simulink model "radar_final_cs_old"  (R2019a)
settings: Solver=ode5  StartTime=0.0  StopTime=2  FixedStep=1/20  RelTol=1e-3
PreLoadFcn:
  | mbxruntime.callbacks.PreLoadFcn(bdroot);
PostLoadFcn:
  | mbxruntime.callbacks.PostLoadFcn(bdroot);
InitFcn:
  | mbxruntime.callbacks.InitFcn(bdroot);
StartFcn:
  | mbxruntime.callbacks.StartFcn(bdroot);
StopFcn:
  | mbxruntime.callbacks.StopFcn(bdroot);
model workspace: external: MAT-File .\radar_final_cs_hws.mat (data not in the file)
undefined symbols (not defined in the file or in its folder): Data, Data_SL_Info, DiscIntNeverNeededParam, mbxruntime, radar_final_cs_06f3e03c41833990, radar_final_cs_0ae852e737f0605d, radar_final_cs_2161ee680ff58ba6, radar_final_cs_2267e09559a0c517, radar_final_cs_25fb437f13dc4ac4, radar_final_cs_2a9ff95eb5b29c63, radar_final_cs_2b3b1caad78d25a0, radar_final_cs_36e6d5e535f2778e, radar_final_cs_3f094c3a86d4ef6f, radar_final_cs_414d34a7c1c059ce, radar_final_cs_42788e9f25b76679, radar_final_cs_4442007d7943b1b9, radar_final_cs_57cb0909d4e1963a, radar_final_cs_647e288b34857263, radar_final_cs_7d2d9604fce16766, radar_final_cs_898d5fa4c0c4dce2, radar_final_cs_a56cd948251ec351, radar_final_cs_Audi_A3_2_Path_pathUniqueID, radar_final_cs_Audi_A3_2_SpeedProfile_speedProfileUniqueID, radar_final_cs_bc1d53445e794831, radar_final_cs_bc84f0b4aab11bdd, radar_final_cs_bd2c14ed7a8a21e4, radar_final_cs_bdb595cdc91a90da, radar_final_cs_Boy_150_1_Dynamics_Empty_STATE_Boy_150_1_Pitch0, radar_final_cs_Boy_150_1_Dynamics_Empty_STATE_Boy_150_1_Roll0, radar_final_cs_Boy_150_1_Dynamics_Empty_STATE_Boy_150_1_x0, radar_final_cs_Boy_150_1_Dynamics_Empty_STATE_Boy_150_1_y0, radar_final_cs_Boy_150_1_Dynamics_Empty_STATE_Boy_150_1_Yaw0, radar_final_cs_Boy_150_1_Dynamics_Empty_STATE_Boy_150_1_z0, radar_final_cs_c30ea0c83d921ad6, radar_final_cs_c7f661c76d99b58c, radar_final_cs_ce7e016dbedf2c74, radar_final_cs_cf2ef22c3980d47c, radar_final_cs_d0ac9bfbee56c7a8, radar_final_cs_d13fb20b651cdee7, radar_final_cs_da52fa0c45f9873a, radar_final_cs_f7605f9552b276d3, radar_final_cs_ff9f13297006dd64, radar_final_cs_Skywell_1_Path_pathUniqueID, radar_final_cs_Skywell_1_SpeedProfile_speedProfileUniqueID, tabledata, X, Y
libraries: PreScanSimulinkLibrary x12, simulink x7, robotlib x5, PreScanUsefulBlocks x1
(part 3 of 5)

== system radar_final_cs_old/STATE_Male_Female_HandInHand_1_bus ==
  STATE_Male_Female_HandInHand_1_bus : Inport  Tag=inport/StatePort  OutDataTypeStr=Bus: PRESCAN_STATEACTUATORDATA  PortDimensions=1  SampleTime=1/20  BusOutputAsStruct=on
  Actuator : S-Function  FunctionName=sfun_StateActuator  Parameters=mbxruntime.parameters.convert(UniqueID), mbxruntime.parameters.convert(TimeStep)  SFunctionDeploymentMode=off  EnableBusSupport=off  mask(PreScan Sink Block: State){UniqueID=523, TimeStep=1/20}
      mask prompts: UniqueID "Auto-Assigned: Unique ID"; TimeStep "Auto-Assigned: Upload Period [s]"
      mask help:
      | The Actor State contains a vector signal of size (9x1), containing the following signals:
      |
      | -  Position    	(x,y,z)             	[m]
      | -  Velocity    	(vx,vy,vz)         	[m/s]
      | -  Angles       	(Roll, Pitch, Yaw)	[rad]
      |
      | The Actor state is defined in the global axis system.
      | The state is superponed on the Initial position defined in the GUI.
      |
      | For more information, please click Help.
      mask Help: eval('openHelp(222)')
      mask Display: image(imread('State.png'))
  wires:
  STATE_Male_Female_HandInHand_1_bus/1 -> Actuator/1

== system radar_final_cs_old/STATE_Skywell_1_bus ==
  STATE_Skywell_1_bus : Inport  Tag=inport/StatePort  OutDataTypeStr=Bus: PRESCAN_STATEACTUATORDATA  PortDimensions=1  SampleTime=1/20  BusOutputAsStruct=on
  Actuator : S-Function  FunctionName=sfun_StateActuator  Parameters=mbxruntime.parameters.convert(UniqueID), mbxruntime.parameters.convert(TimeStep)  SFunctionDeploymentMode=off  EnableBusSupport=off  mask(PreScan Sink Block: State){UniqueID=169, TimeStep=1/20}
      mask prompts: UniqueID "Auto-Assigned: Unique ID"; TimeStep "Auto-Assigned: Upload Period [s]"
      mask help:
      | The Actor State contains a vector signal of size (9x1), containing the following signals:
      |
      | -  Position    	(x,y,z)             	[m]
      | -  Velocity    	(vx,vy,vz)         	[m/s]
      | -  Angles       	(Roll, Pitch, Yaw)	[rad]
      |
      | The Actor state is defined in the global axis system.
      | The state is superponed on the Initial position defined in the GUI.
      |
      | For more information, please click Help.
      mask Help: eval('openHelp(222)')
      mask Display: image(imread('State.png'))
  wires:
  STATE_Skywell_1_bus/1 -> Actuator/1

== system radar_final_cs_old/ScenarioEngine ==
  Clock1 : Clock
  Stop Simulation : Stop
  sfun_ScenarioEngine1 : S-Function  FunctionName=sfun_ScenarioEngine  Parameters=TimeStep  SFunctionDeploymentMode=off  EnableBusSupport=off
  wires:
  sfun_ScenarioEngine1/1 -> Stop Simulation/1
  Clock1/1 -> sfun_ScenarioEngine1/1

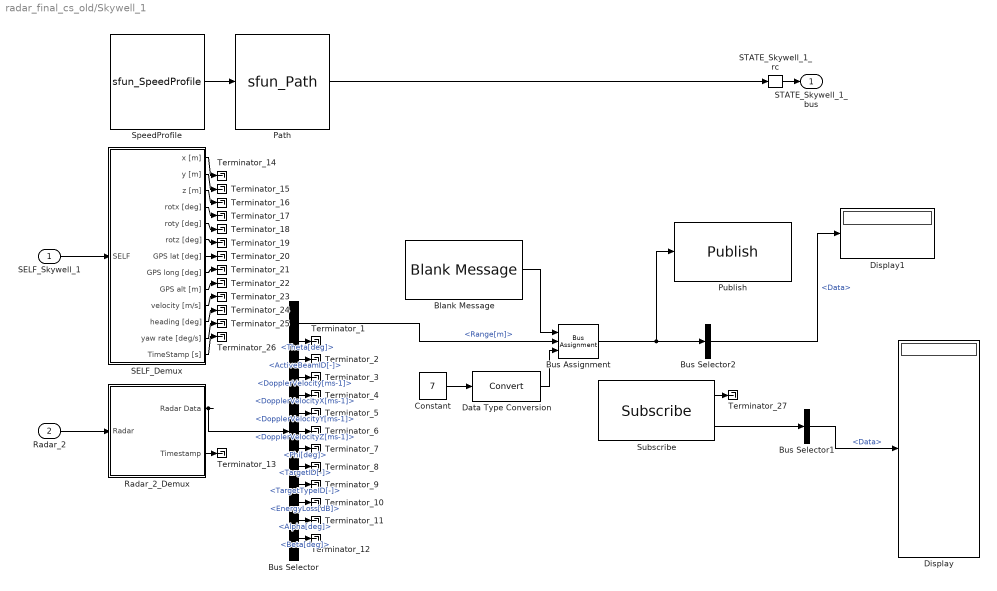
== system radar_final_cs_old/Skywell_1 ==
  SELF_Skywell_1 : Inport  Tag=inport/SelfPort  OutDataTypeStr=Bus: PRESCAN_SELFSENSORDATA  PortDimensions=1  SampleTime=1/20  BusOutputAsStruct=on
  Radar_2 : Inport  Tag=inport/Radar  Port=2  OutDataTypeStr=Bus: PRESCAN_SCANNERSENSOR_MESSAGE  PortDimensions=7  SampleTime=1/4  BusOutputAsStruct=on
  Blank Message : robotlib/Blank Message  messageClass=Message  entityType=std_msgs/Float64MultiArray  messageType=std_msgs/Float64MultiArray  SampleTime=inf
      settings: SourceProductBaseCode=RO
  Bus Assignment : BusAssignment  AssignedSignals=Data,Data_SL_Info.CurrentLength
  Bus Selector : BusSelector  OutputSignals=Range[m],Theta[deg],ActiveBeamID[-],DopplerVelocity[ms-1],DopplerVelocityX[ms-1],DopplerVelocityY[ms-1],DopplerVelocityZ[ms-1],Phi[deg],TargetID[-],TargetTypeID[-],EnergyLoss[dB],Alpha[deg],Beta[deg]
  Bus Selector1 : BusSelector  OutputSignals=Data
  Bus Selector2 : BusSelector  OutputSignals=Data
  Constant : Constant  Value=7
  Data Type Conversion : DataTypeConversion
  Display : Display
  Display1 : Display
  Path : S-Function  LoadFcn=load('PrescanMotionData.mat')  FunctionName=sfun_Path  Parameters=mbxruntime.parameters.convert(uniqueID), pathUniqueID, mbxruntime.parameters.convert(timestep)  SFunctionDeploymentMode=off  EnableBusSupport=off  mask(Path){uniqueID=169, pathUniqueID=radar_final_cs_Skywell_1_Path_pathUniqueID, timestep=1/20}
      mask prompts: uniqueID "Object Unique ID"; pathUniqueID "Path Unique ID"; timestep "MATLAB timestep:"
      mask help:
      | The path block outputs the position along a given trajectory.
      |
      | For more information, please click Help.
      mask Help: eval('openHelp(312)')
      mask Display: image(imread('Path.png'))
  Publish : robotlib/Publish  topicSource=Specify your own  topic=/topic  messageType=std_msgs/Float64MultiArray  messageQueueLength=1
      settings: SourceProductBaseCode=RO
  Radar_2_Demux : Subsystem  Tag=demux/Radar  TreatAsAtomicUnit=on  mask(PreScan Demux Block: Radar){MAXMESSAGES=7}
      mask prompts: MAXMESSAGES "Number of Objects"
      mask help:
      | The Radar Sensor is a detailed sensor based on a physical radar
      | model that includes Antenna GAIN Maps (AGM) and atmospheric
      | attenuation.
      |
      | For more information, please click Help.
      mask Help: eval('openHelp(1464)')
      mask Display:
      | port_label('input',1,'Radar')
      | port_label('output',1,'Radar Data')
      | port_label('output',2,'Timestamp [s]')
  SELF_Demux : Subsystem  Tag=demux/SelfPort  mask(PreScan Demux Block:){}
      mask help:
      | The SELF port shows (state) information of the actor itself. The outputs are position in the experiment's axis system and the GPS coordinates, and the object's absolute velocity and compass heading.
      |
      | For more information, please click Help.
      settings: DeleteFcn=PreScanBlockDeleteFcn;
      mask Help: eval('openHelp(462)')
      mask Display:
      | port_label('output',1,'x [m]')
      | port_label('output',2,'y [m]')
      | port_label('output',3,'z [m]','texmode','on')
      | port_label('output',4,'Rotx [deg]','texmode','on')
      | port_label('output',5,'Roty [deg]','texmode','on')
      | port_label('output',6,'Rotz [deg]','texmode','on')
      | port_label('output',7,'GPS lat [deg]','texmode','on')
      | port_label('output',8,'GPS long [deg]','texmode','on')
      | port_label('output',9,'GPS alt [m]','texmode','on')
      | port_label('output',10,'Velocity [m/s]')
      | port_label('output',11,'Heading [deg]')
      | port_label('output',12,'Yaw rate [deg/s]')
      | port_label('output',13,'Timestamp [s]')
  STATE_Skywell_1_rc : RateTransition  Tag=mux_rc/StatePort  OutPortSampleTimeOpt=Inherit
  SpeedProfile : S-Function  LoadFcn=load('PrescanMotionData.mat')  FunctionName=sfun_SpeedProfile  Parameters=speedProfileUniqueID, mbxruntime.parameters.convert(timestep)  SFunctionDeploymentMode=off  EnableBusSupport=off  mask(SpeedProfile){speedProfileUniqueID=radar_final_cs_Skywell_1_SpeedProfile_speedProfileUniqueID, timestep=1/20}
      mask prompts: speedProfileUniqueID "Speed Profile Unique ID"; timestep "MATLAB timestep:"
      mask help:
      | The speed profile block outputs the travelled distance, velocities and acceleration along a given path.
      |
      | For more information, please click Help.
      mask Help: eval('openHelp(312)')
      mask Display: image(imread('SpeedProfile.png'))
  Subscribe : robotlib/Subscribe  topicSource=Specify your own  topic=/topic  messageType=std_msgs/Float64MultiArray  sampleTime=-1  messageQueueLength=1
      settings: SourceProductBaseCode=RO
  Terminator_{1..27} (27 alike) : Terminator
  STATE_Skywell_1_bus : Outport  Tag=outport/StatePort  OutDataTypeStr=Bus: PRESCAN_STATEACTUATORDATA  PortDimensions=1  SampleTime=1/20
  wires:
  Radar_2_Demux/1(Radar Data) -> Bus Selector/1
  Blank Message/1 -> Bus Assignment/1
  Bus Selector/1 -> Bus Assignment/2  "<Range[m]>"
  Bus Assignment/1 -> Publish/1, Bus Selector2/1
  Subscribe/2 -> Bus Selector1/1
  Bus Selector1/1 -> Display/1  "<Data>"
  Bus Selector2/1 -> Display1/1  "<Data>"
  Data Type Conversion/1 -> Bus Assignment/3
  Constant/1 -> Data Type Conversion/1
  STATE_Skywell_1_rc/1 -> STATE_Skywell_1_bus/1
  SpeedProfile/1 -> Path/1
  Path/1 -> STATE_Skywell_1_rc/1
  SELF_Skywell_1/1 -> SELF_Demux/1(SELF)
  Radar_2/1 -> Radar_2_Demux/1(Radar)
  Bus Selector/2 -> Terminator_1/1  "<Theta[deg]>"
  Bus Selector/3 -> Terminator_2/1  "<ActiveBeamID[-]>"
  Bus Selector/4 -> Terminator_3/1  "<DopplerVelocity[ms-1]>"
  Bus Selector/5 -> Terminator_4/1  "<DopplerVelocityX[ms-1]>"
  Bus Selector/6 -> Terminator_5/1  "<DopplerVelocityY[ms-1]>"
  Bus Selector/7 -> Terminator_6/1  "<DopplerVelocityZ[ms-1]>"
  Bus Selector/8 -> Terminator_7/1  "<Phi[deg]>"
  Bus Selector/9 -> Terminator_8/1  "<TargetID[-]>"
  Bus Selector/10 -> Terminator_9/1  "<TargetTypeID[-]>"
  Bus Selector/11 -> Terminator_10/1  "<EnergyLoss[dB]>"
  Bus Selector/12 -> Terminator_11/1  "<Alpha[deg]>"
  Bus Selector/13 -> Terminator_12/1  "<Beta[deg]>"
  Radar_2_Demux/2(Timestamp) -> Terminator_13/1
  SELF_Demux/1(x [m]) -> Terminator_14/1
  SELF_Demux/2(y [m]) -> Terminator_15/1
  SELF_Demux/3(z [m]) -> Terminator_16/1
  SELF_Demux/4(rotx [deg]) -> Terminator_17/1
  SELF_Demux/5(roty [deg]) -> Terminator_18/1
  SELF_Demux/6(rotz [deg]) -> Terminator_19/1
  SELF_Demux/7(GPS lat [deg]) -> Terminator_20/1
  SELF_Demux/8(GPS long [deg]) -> Terminator_21/1
  SELF_Demux/9(GPS alt [m]) -> Terminator_22/1
  SELF_Demux/10(velocity [m/s]) -> Terminator_23/1
  SELF_Demux/11(heading [deg]) -> Terminator_24/1
  SELF_Demux/12(yaw rate [deg/s]) -> Terminator_25/1
  SELF_Demux/13(TimeStamp [s]) -> Terminator_26/1
  Subscribe/1 -> Terminator_27/1

== system radar_final_cs_old/Synchronizer ==
  Bus Selector1 : BusSelector  OutputSignals=FederateStopped
  Stop Simulation : Stop
  sfun_Synchronizer : S-Function  FunctionName=sfun_Synchronizer  Parameters=SampleTime  SFunctionDeploymentMode=off  EnableBusSupport=off  mask(Legacy Function){SFunctionSpec=void prescan_synchronizer_outputFcn(void ** work1, PRESCAN_SYNCHRONIZEDATA y1[1]), SampleTime=TimeStep, ShowSpec=on}
      mask prompts: SampleTime "Sample time (-1 for inherited):"; ShowSpec "Display function specification"
      mask help:
      | This block allows you to call the legacy functions specified by the following Legacy Code Tool definition:
      | def.SFunctionName = 'sfun_Synchronizer';
      | def.OutputFcnSpec = 'void prescan_synchronizer_outputFcn(void ** work1, PRESCAN_TIMESTAMPDATA u1[1], PRESCAN_SYNCHRONIZEDATA y1[1])';
      | def.StartFcnSpec = 'void prescan_synchronizer_startFcn(void ** work1)';
      | def.TerminateFcnSpec = 'void prescan_synchronizer_terminateFcn(void ** work1)';
      | def.HeaderFiles = {'prescan_synchronizer_data.h'};
      | def.HostLibFiles = {'sensorinterfaced.lib'};
      | def.IncPaths = {'src', 'C:\prescandev\vislibrary\vis\..\pimp\include\sensors\InterfaceRTW'};
      | def.SrcPaths = {'src'};
      | def.LibPaths = {'C:\\prescandev\\vislibrary_build\lib'};
      | def.SampleTime = 'parameterized';
      | def.Options.language = 'C';
      mask Help: <p>This block was generated automatically by the Legacy Code Tool. For detailed help on this tool, call<a href="matlab:legacy_code('help')"> legacy_code('help')</a>.</p>
      mask Callback ShowSpec:
      | if strcmp(get_param(gcbh, 'ShowSpec'), 'on')
      |   set_param(gcbh, 'MaskDisplay', sprintf('fprintf(''%s'');', get_param(gcbh, 'SFunctionSpec')));
      | else
      |   set_param(gcbh, 'MaskDisplay', sprintf('fprintf(''%s'');', get_param(gcbh, 'FunctionName')));
      | end
      mask Display: fprintf('void prescan_synchronizer_outputFcn(void ** work1, PRESCAN_SYNCHRONIZEDATA y1[1])');
  wires:
  sfun_Synchronizer/1 -> Bus Selector1/1
  Bus Selector1/1 -> Stop Simulation/1  "<FederateStopped>"

== system radar_final_cs_old/VISUColorRegion_Lower_Body_Boy_150_1 ==
  VISUColorRegion_Lower_Body_Boy_150_1 : Inport  Tag=inport/ColorRegion  OutDataTypeStr=Bus: PRESCAN_COLOR_DATA  PortDimensions=1  SampleTime=1/20  BusOutputAsStruct=on
  Actuator : S-Function  FunctionName=sfun_ColorActuator  Parameters=mbxruntime.parameters.convert(UniqueID), mbxruntime.parameters.convert(WorldModelSubPath), tabledata, TimeStep  SFunctionDeploymentMode=off  EnableBusSupport=off  mask(PreScan Sink Block: VisuTextureColor){UniqueID=197, WorldModelSubPath=/recolorRegion:name=Lower Body/targetColor, TimeStep=1/20}
      mask prompts: UniqueID "Parent Unique Identifier (auto-generated)"; WorldModelSubPath "WM SubPath(auto-generated)"; TimeStep "Simulink time step"
      mask help:
      | The VisuTextureColor block provides a way to adapt the color of a vehicle.
      |
      | For more information, please click Help.
      mask init:
      | [tabledata] = mbxruntime.parameters.table(UniqueID,WorldModelSubPath);
      mask Help: eval('openHelp(230)')
      mask Display: image(imread('TextureColor.png'))
  wires:
  VISUColorRegion_Lower_Body_Boy_150_1/1 -> Actuator/1

== system radar_final_cs_old/VISUColorRegion_Lower_Body_Child_Leaning_1 ==
  VISUColorRegion_Lower_Body_Child_Leaning_1 : Inport  Tag=inport/ColorRegion  OutDataTypeStr=Bus: PRESCAN_COLOR_DATA  PortDimensions=1  SampleTime=1/20  BusOutputAsStruct=on
  Actuator : S-Function  FunctionName=sfun_ColorActuator  Parameters=mbxruntime.parameters.convert(UniqueID), mbxruntime.parameters.convert(WorldModelSubPath), tabledata, TimeStep  SFunctionDeploymentMode=off  EnableBusSupport=off  mask(PreScan Sink Block: VisuTextureColor){UniqueID=387, WorldModelSubPath=/recolorRegion:name=Lower Body/targetColor, TimeStep=1/20}
      mask prompts: UniqueID "Parent Unique Identifier (auto-generated)"; WorldModelSubPath "WM SubPath(auto-generated)"; TimeStep "Simulink time step"
      mask help:
      | The VisuTextureColor block provides a way to adapt the color of a vehicle.
      |
      | For more information, please click Help.
      mask init:
      | [tabledata] = mbxruntime.parameters.table(UniqueID,WorldModelSubPath);
      mask Help: eval('openHelp(230)')
      mask Display: image(imread('TextureColor.png'))
  wires:
  VISUColorRegion_Lower_Body_Child_Leaning_1/1 -> Actuator/1

== system radar_final_cs_old/VISUColorRegion_Lower_Body_Child_Overweight_1 ==
  VISUColorRegion_Lower_Body_Child_Overweight_1 : Inport  Tag=inport/ColorRegion  OutDataTypeStr=Bus: PRESCAN_COLOR_DATA  PortDimensions=1  SampleTime=1/20  BusOutputAsStruct=on
  Actuator : S-Function  FunctionName=sfun_ColorActuator  Parameters=mbxruntime.parameters.convert(UniqueID), mbxruntime.parameters.convert(WorldModelSubPath), tabledata, TimeStep  SFunctionDeploymentMode=off  EnableBusSupport=off  mask(PreScan Sink Block: VisuTextureColor){UniqueID=388, WorldModelSubPath=/recolorRegion:name=Lower Body/targetColor, TimeStep=1/20}
      mask prompts: UniqueID "Parent Unique Identifier (auto-generated)"; WorldModelSubPath "WM SubPath(auto-generated)"; TimeStep "Simulink time step"
      mask help:
      | The VisuTextureColor block provides a way to adapt the color of a vehicle.
      |
      | For more information, please click Help.
      mask init:
      | [tabledata] = mbxruntime.parameters.table(UniqueID,WorldModelSubPath);
      mask Help: eval('openHelp(230)')
      mask Display: image(imread('TextureColor.png'))
  wires:
  VISUColorRegion_Lower_Body_Child_Overweight_1/1 -> Actuator/1

== system radar_final_cs_old/VISUColorRegion_Lower_Body_Child_Regular_1 ==
  VISUColorRegion_Lower_Body_Child_Regular_1 : Inport  Tag=inport/ColorRegion  OutDataTypeStr=Bus: PRESCAN_COLOR_DATA  PortDimensions=1  SampleTime=1/20  BusOutputAsStruct=on
  Actuator : S-Function  FunctionName=sfun_ColorActuator  Parameters=mbxruntime.parameters.convert(UniqueID), mbxruntime.parameters.convert(WorldModelSubPath), tabledata, TimeStep  SFunctionDeploymentMode=off  EnableBusSupport=off  mask(PreScan Sink Block: VisuTextureColor){UniqueID=389, WorldModelSubPath=/recolorRegion:name=Lower Body/targetColor, TimeStep=1/20}
      mask prompts: UniqueID "Parent Unique Identifier (auto-generated)"; WorldModelSubPath "WM SubPath(auto-generated)"; TimeStep "Simulink time step"
      mask help:
      | The VisuTextureColor block provides a way to adapt the color of a vehicle.
      |
      | For more information, please click Help.
      mask init:
      | [tabledata] = mbxruntime.parameters.table(UniqueID,WorldModelSubPath);
      mask Help: eval('openHelp(230)')
      mask Display: image(imread('TextureColor.png'))
  wires:
  VISUColorRegion_Lower_Body_Child_Regular_1/1 -> Actuator/1

== system radar_final_cs_old/VISUColorRegion_Lower_Body_Child_Regular_2 ==
  VISUColorRegion_Lower_Body_Child_Regular_2 : Inport  Tag=inport/ColorRegion  OutDataTypeStr=Bus: PRESCAN_COLOR_DATA  PortDimensions=1  SampleTime=1/20  BusOutputAsStruct=on
  Actuator : S-Function  FunctionName=sfun_ColorActuator  Parameters=mbxruntime.parameters.convert(UniqueID), mbxruntime.parameters.convert(WorldModelSubPath), tabledata, TimeStep  SFunctionDeploymentMode=off  EnableBusSupport=off  mask(PreScan Sink Block: VisuTextureColor){UniqueID=390, WorldModelSubPath=/recolorRegion:name=Lower Body/targetColor, TimeStep=1/20}
      mask prompts: UniqueID "Parent Unique Identifier (auto-generated)"; WorldModelSubPath "WM SubPath(auto-generated)"; TimeStep "Simulink time step"
      mask help:
      | The VisuTextureColor block provides a way to adapt the color of a vehicle.
      |
      | For more information, please click Help.
      mask init:
      | [tabledata] = mbxruntime.parameters.table(UniqueID,WorldModelSubPath);
      mask Help: eval('openHelp(230)')
      mask Display: image(imread('TextureColor.png'))
  wires:
  VISUColorRegion_Lower_Body_Child_Regular_2/1 -> Actuator/1

== system radar_final_cs_old/VISUColorRegion_Lower_Body_Male_Female_HandInHand_1 ==
  VISUColorRegion_Lower_Body_Male_Female_HandInHand_1 : Inport  Tag=inport/ColorRegion  OutDataTypeStr=Bus: PRESCAN_COLOR_DATA  PortDimensions=1  SampleTime=1/20  BusOutputAsStruct=on
  Actuator : S-Function  FunctionName=sfun_ColorActuator  Parameters=mbxruntime.parameters.convert(UniqueID), mbxruntime.parameters.convert(WorldModelSubPath), tabledata, TimeStep  SFunctionDeploymentMode=off  EnableBusSupport=off  mask(PreScan Sink Block: VisuTextureColor){UniqueID=523, WorldModelSubPath=/recolorRegion:name=Lower Body/targetColor, TimeStep=1/20}
      mask prompts: UniqueID "Parent Unique Identifier (auto-generated)"; WorldModelSubPath "WM SubPath(auto-generated)"; TimeStep "Simulink time step"
      mask help:
      | The VisuTextureColor block provides a way to adapt the color of a vehicle.
      |
      | For more information, please click Help.
      mask init:
      | [tabledata] = mbxruntime.parameters.table(UniqueID,WorldModelSubPath);
      mask Help: eval('openHelp(230)')
      mask Display: image(imread('TextureColor.png'))
  wires:
  VISUColorRegion_Lower_Body_Male_Female_HandInHand_1/1 -> Actuator/1

== system radar_final_cs_old/VISUColorRegion_Shoes_Boy_150_1 ==
  VISUColorRegion_Shoes_Boy_150_1 : Inport  Tag=inport/ColorRegion  OutDataTypeStr=Bus: PRESCAN_COLOR_DATA  PortDimensions=1  SampleTime=1/20  BusOutputAsStruct=on
  Actuator : S-Function  FunctionName=sfun_ColorActuator  Parameters=mbxruntime.parameters.convert(UniqueID), mbxruntime.parameters.convert(WorldModelSubPath), tabledata, TimeStep  SFunctionDeploymentMode=off  EnableBusSupport=off  mask(PreScan Sink Block: VisuTextureColor){UniqueID=197, WorldModelSubPath=/recolorRegion:name=Shoes/targetColor, TimeStep=1/20}
      mask prompts: UniqueID "Parent Unique Identifier (auto-generated)"; WorldModelSubPath "WM SubPath(auto-generated)"; TimeStep "Simulink time step"
      mask help:
      | The VisuTextureColor block provides a way to adapt the color of a vehicle.
      |
      | For more information, please click Help.
      mask init:
      | [tabledata] = mbxruntime.parameters.table(UniqueID,WorldModelSubPath);
      mask Help: eval('openHelp(230)')
      mask Display: image(imread('TextureColor.png'))
  wires:
  VISUColorRegion_Shoes_Boy_150_1/1 -> Actuator/1

== system radar_final_cs_old/VISUColorRegion_Shoes_Child_Leaning_1 ==
  VISUColorRegion_Shoes_Child_Leaning_1 : Inport  Tag=inport/ColorRegion  OutDataTypeStr=Bus: PRESCAN_COLOR_DATA  PortDimensions=1  SampleTime=1/20  BusOutputAsStruct=on
  Actuator : S-Function  FunctionName=sfun_ColorActuator  Parameters=mbxruntime.parameters.convert(UniqueID), mbxruntime.parameters.convert(WorldModelSubPath), tabledata, TimeStep  SFunctionDeploymentMode=off  EnableBusSupport=off  mask(PreScan Sink Block: VisuTextureColor){UniqueID=387, WorldModelSubPath=/recolorRegion:name=Shoes/targetColor, TimeStep=1/20}
      mask prompts: UniqueID "Parent Unique Identifier (auto-generated)"; WorldModelSubPath "WM SubPath(auto-generated)"; TimeStep "Simulink time step"
      mask help:
      | The VisuTextureColor block provides a way to adapt the color of a vehicle.
      |
      | For more information, please click Help.
      mask init:
      | [tabledata] = mbxruntime.parameters.table(UniqueID,WorldModelSubPath);
      mask Help: eval('openHelp(230)')
      mask Display: image(imread('TextureColor.png'))
  wires:
  VISUColorRegion_Shoes_Child_Leaning_1/1 -> Actuator/1

== system radar_final_cs_old/VISUColorRegion_Shoes_Child_Overweight_1 ==
  VISUColorRegion_Shoes_Child_Overweight_1 : Inport  Tag=inport/ColorRegion  OutDataTypeStr=Bus: PRESCAN_COLOR_DATA  PortDimensions=1  SampleTime=1/20  BusOutputAsStruct=on
  Actuator : S-Function  FunctionName=sfun_ColorActuator  Parameters=mbxruntime.parameters.convert(UniqueID), mbxruntime.parameters.convert(WorldModelSubPath), tabledata, TimeStep  SFunctionDeploymentMode=off  EnableBusSupport=off  mask(PreScan Sink Block: VisuTextureColor){UniqueID=388, WorldModelSubPath=/recolorRegion:name=Shoes/targetColor, TimeStep=1/20}
      mask prompts: UniqueID "Parent Unique Identifier (auto-generated)"; WorldModelSubPath "WM SubPath(auto-generated)"; TimeStep "Simulink time step"
      mask help:
      | The VisuTextureColor block provides a way to adapt the color of a vehicle.
      |
      | For more information, please click Help.
      mask init:
      | [tabledata] = mbxruntime.parameters.table(UniqueID,WorldModelSubPath);
      mask Help: eval('openHelp(230)')
      mask Display: image(imread('TextureColor.png'))
  wires:
  VISUColorRegion_Shoes_Child_Overweight_1/1 -> Actuator/1

== system radar_final_cs_old/VISUColorRegion_Shoes_Child_Regular_1 ==
  VISUColorRegion_Shoes_Child_Regular_1 : Inport  Tag=inport/ColorRegion  OutDataTypeStr=Bus: PRESCAN_COLOR_DATA  PortDimensions=1  SampleTime=1/20  BusOutputAsStruct=on
  Actuator : S-Function  FunctionName=sfun_ColorActuator  Parameters=mbxruntime.parameters.convert(UniqueID), mbxruntime.parameters.convert(WorldModelSubPath), tabledata, TimeStep  SFunctionDeploymentMode=off  EnableBusSupport=off  mask(PreScan Sink Block: VisuTextureColor){UniqueID=389, WorldModelSubPath=/recolorRegion:name=Shoes/targetColor, TimeStep=1/20}
      mask prompts: UniqueID "Parent Unique Identifier (auto-generated)"; WorldModelSubPath "WM SubPath(auto-generated)"; TimeStep "Simulink time step"
      mask help:
      | The VisuTextureColor block provides a way to adapt the color of a vehicle.
      |
      | For more information, please click Help.
      mask init:
      | [tabledata] = mbxruntime.parameters.table(UniqueID,WorldModelSubPath);
      mask Help: eval('openHelp(230)')
      mask Display: image(imread('TextureColor.png'))
  wires:
  VISUColorRegion_Shoes_Child_Regular_1/1 -> Actuator/1

== system radar_final_cs_old/VISUColorRegion_Shoes_Child_Regular_2 ==
  VISUColorRegion_Shoes_Child_Regular_2 : Inport  Tag=inport/ColorRegion  OutDataTypeStr=Bus: PRESCAN_COLOR_DATA  PortDimensions=1  SampleTime=1/20  BusOutputAsStruct=on
  Actuator : S-Function  FunctionName=sfun_ColorActuator  Parameters=mbxruntime.parameters.convert(UniqueID), mbxruntime.parameters.convert(WorldModelSubPath), tabledata, TimeStep  SFunctionDeploymentMode=off  EnableBusSupport=off  mask(PreScan Sink Block: VisuTextureColor){UniqueID=390, WorldModelSubPath=/recolorRegion:name=Shoes/targetColor, TimeStep=1/20}
      mask prompts: UniqueID "Parent Unique Identifier (auto-generated)"; WorldModelSubPath "WM SubPath(auto-generated)"; TimeStep "Simulink time step"
      mask help:
      | The VisuTextureColor block provides a way to adapt the color of a vehicle.
      |
      | For more information, please click Help.
      mask init:
      | [tabledata] = mbxruntime.parameters.table(UniqueID,WorldModelSubPath);
      mask Help: eval('openHelp(230)')
      mask Display: image(imread('TextureColor.png'))
  wires:
  VISUColorRegion_Shoes_Child_Regular_2/1 -> Actuator/1

== system radar_final_cs_old/VISUColorRegion_Shoes_Male_Female_HandInHand_1 ==
  VISUColorRegion_Shoes_Male_Female_HandInHand_1 : Inport  Tag=inport/ColorRegion  OutDataTypeStr=Bus: PRESCAN_COLOR_DATA  PortDimensions=1  SampleTime=1/20  BusOutputAsStruct=on
  Actuator : S-Function  FunctionName=sfun_ColorActuator  Parameters=mbxruntime.parameters.convert(UniqueID), mbxruntime.parameters.convert(WorldModelSubPath), tabledata, TimeStep  SFunctionDeploymentMode=off  EnableBusSupport=off  mask(PreScan Sink Block: VisuTextureColor){UniqueID=523, WorldModelSubPath=/recolorRegion:name=Shoes/targetColor, TimeStep=1/20}
      mask prompts: UniqueID "Parent Unique Identifier (auto-generated)"; WorldModelSubPath "WM SubPath(auto-generated)"; TimeStep "Simulink time step"
      mask help:
      | The VisuTextureColor block provides a way to adapt the color of a vehicle.
      |
      | For more information, please click Help.
      mask init:
      | [tabledata] = mbxruntime.parameters.table(UniqueID,WorldModelSubPath);
      mask Help: eval('openHelp(230)')
      mask Display: image(imread('TextureColor.png'))
  wires:
  VISUColorRegion_Shoes_Male_Female_HandInHand_1/1 -> Actuator/1

== system radar_final_cs_old/VISUColorRegion_Upper_Body_Boy_150_1 ==
  VISUColorRegion_Upper_Body_Boy_150_1 : Inport  Tag=inport/ColorRegion  OutDataTypeStr=Bus: PRESCAN_COLOR_DATA  PortDimensions=1  SampleTime=1/20  BusOutputAsStruct=on
  Actuator : S-Function  FunctionName=sfun_ColorActuator  Parameters=mbxruntime.parameters.convert(UniqueID), mbxruntime.parameters.convert(WorldModelSubPath), tabledata, TimeStep  SFunctionDeploymentMode=off  EnableBusSupport=off  mask(PreScan Sink Block: VisuTextureColor){UniqueID=197, WorldModelSubPath=/recolorRegion:name=Upper Body/targetColor, TimeStep=1/20}
      mask prompts: UniqueID "Parent Unique Identifier (auto-generated)"; WorldModelSubPath "WM SubPath(auto-generated)"; TimeStep "Simulink time step"
      mask help:
      | The VisuTextureColor block provides a way to adapt the color of a vehicle.
      |
      | For more information, please click Help.
      mask init:
      | [tabledata] = mbxruntime.parameters.table(UniqueID,WorldModelSubPath);
      mask Help: eval('openHelp(230)')
      mask Display: image(imread('TextureColor.png'))
  wires:
  VISUColorRegion_Upper_Body_Boy_150_1/1 -> Actuator/1

== system radar_final_cs_old/VISUColorRegion_Upper_Body_Child_Leaning_1 ==
  VISUColorRegion_Upper_Body_Child_Leaning_1 : Inport  Tag=inport/ColorRegion  OutDataTypeStr=Bus: PRESCAN_COLOR_DATA  PortDimensions=1  SampleTime=1/20  BusOutputAsStruct=on
  Actuator : S-Function  FunctionName=sfun_ColorActuator  Parameters=mbxruntime.parameters.convert(UniqueID), mbxruntime.parameters.convert(WorldModelSubPath), tabledata, TimeStep  SFunctionDeploymentMode=off  EnableBusSupport=off  mask(PreScan Sink Block: VisuTextureColor){UniqueID=387, WorldModelSubPath=/recolorRegion:name=Upper Body/targetColor, TimeStep=1/20}
      mask prompts: UniqueID "Parent Unique Identifier (auto-generated)"; WorldModelSubPath "WM SubPath(auto-generated)"; TimeStep "Simulink time step"
      mask help:
      | The VisuTextureColor block provides a way to adapt the color of a vehicle.
      |
      | For more information, please click Help.
      mask init:
      | [tabledata] = mbxruntime.parameters.table(UniqueID,WorldModelSubPath);
      mask Help: eval('openHelp(230)')
      mask Display: image(imread('TextureColor.png'))
  wires:
  VISUColorRegion_Upper_Body_Child_Leaning_1/1 -> Actuator/1

== system radar_final_cs_old/VISUColorRegion_Upper_Body_Child_Overweight_1 ==
  VISUColorRegion_Upper_Body_Child_Overweight_1 : Inport  Tag=inport/ColorRegion  OutDataTypeStr=Bus: PRESCAN_COLOR_DATA  PortDimensions=1  SampleTime=1/20  BusOutputAsStruct=on
  Actuator : S-Function  FunctionName=sfun_ColorActuator  Parameters=mbxruntime.parameters.convert(UniqueID), mbxruntime.parameters.convert(WorldModelSubPath), tabledata, TimeStep  SFunctionDeploymentMode=off  EnableBusSupport=off  mask(PreScan Sink Block: VisuTextureColor){UniqueID=388, WorldModelSubPath=/recolorRegion:name=Upper Body/targetColor, TimeStep=1/20}
      mask prompts: UniqueID "Parent Unique Identifier (auto-generated)"; WorldModelSubPath "WM SubPath(auto-generated)"; TimeStep "Simulink time step"
      mask help:
      | The VisuTextureColor block provides a way to adapt the color of a vehicle.
      |
      | For more information, please click Help.
      mask init:
      | [tabledata] = mbxruntime.parameters.table(UniqueID,WorldModelSubPath);
      mask Help: eval('openHelp(230)')
      mask Display: image(imread('TextureColor.png'))
  wires:
  VISUColorRegion_Upper_Body_Child_Overweight_1/1 -> Actuator/1

== system radar_final_cs_old/VISUColorRegion_Upper_Body_Child_Regular_1 ==
  VISUColorRegion_Upper_Body_Child_Regular_1 : Inport  Tag=inport/ColorRegion  OutDataTypeStr=Bus: PRESCAN_COLOR_DATA  PortDimensions=1  SampleTime=1/20  BusOutputAsStruct=on
  Actuator : S-Function  FunctionName=sfun_ColorActuator  Parameters=mbxruntime.parameters.convert(UniqueID), mbxruntime.parameters.convert(WorldModelSubPath), tabledata, TimeStep  SFunctionDeploymentMode=off  EnableBusSupport=off  mask(PreScan Sink Block: VisuTextureColor){UniqueID=389, WorldModelSubPath=/recolorRegion:name=Upper Body/targetColor, TimeStep=1/20}
      mask prompts: UniqueID "Parent Unique Identifier (auto-generated)"; WorldModelSubPath "WM SubPath(auto-generated)"; TimeStep "Simulink time step"
      mask help:
      | The VisuTextureColor block provides a way to adapt the color of a vehicle.
      |
      | For more information, please click Help.
      mask init:
      | [tabledata] = mbxruntime.parameters.table(UniqueID,WorldModelSubPath);
      mask Help: eval('openHelp(230)')
      mask Display: image(imread('TextureColor.png'))
  wires:
  VISUColorRegion_Upper_Body_Child_Regular_1/1 -> Actuator/1

== system radar_final_cs_old/VISUColorRegion_Upper_Body_Child_Regular_2 ==
  VISUColorRegion_Upper_Body_Child_Regular_2 : Inport  Tag=inport/ColorRegion  OutDataTypeStr=Bus: PRESCAN_COLOR_DATA  PortDimensions=1  SampleTime=1/20  BusOutputAsStruct=on
  Actuator : S-Function  FunctionName=sfun_ColorActuator  Parameters=mbxruntime.parameters.convert(UniqueID), mbxruntime.parameters.convert(WorldModelSubPath), tabledata, TimeStep  SFunctionDeploymentMode=off  EnableBusSupport=off  mask(PreScan Sink Block: VisuTextureColor){UniqueID=390, WorldModelSubPath=/recolorRegion:name=Upper Body/targetColor, TimeStep=1/20}
      mask prompts: UniqueID "Parent Unique Identifier (auto-generated)"; WorldModelSubPath "WM SubPath(auto-generated)"; TimeStep "Simulink time step"
      mask help:
      | The VisuTextureColor block provides a way to adapt the color of a vehicle.
      |
      | For more information, please click Help.
      mask init:
      | [tabledata] = mbxruntime.parameters.table(UniqueID,WorldModelSubPath);
      mask Help: eval('openHelp(230)')
      mask Display: image(imread('TextureColor.png'))
  wires:
  VISUColorRegion_Upper_Body_Child_Regular_2/1 -> Actuator/1

== system radar_final_cs_old/VISUColorRegion_Upper_Body_Male_Female_HandInHand_1 ==
  VISUColorRegion_Upper_Body_Male_Female_HandInHand_1 : Inport  Tag=inport/ColorRegion  OutDataTypeStr=Bus: PRESCAN_COLOR_DATA  PortDimensions=1  SampleTime=1/20  BusOutputAsStruct=on
  Actuator : S-Function  FunctionName=sfun_ColorActuator  Parameters=mbxruntime.parameters.convert(UniqueID), mbxruntime.parameters.convert(WorldModelSubPath), tabledata, TimeStep  SFunctionDeploymentMode=off  EnableBusSupport=off  mask(PreScan Sink Block: VisuTextureColor){UniqueID=523, WorldModelSubPath=/recolorRegion:name=Upper Body/targetColor, TimeStep=1/20}
      mask prompts: UniqueID "Parent Unique Identifier (auto-generated)"; WorldModelSubPath "WM SubPath(auto-generated)"; TimeStep "Simulink time step"
      mask help:
      | The VisuTextureColor block provides a way to adapt the color of a vehicle.
      |
      | For more information, please click Help.
      mask init:
      | [tabledata] = mbxruntime.parameters.table(UniqueID,WorldModelSubPath);
      mask Help: eval('openHelp(230)')
      mask Display: image(imread('TextureColor.png'))
  wires:
  VISUColorRegion_Upper_Body_Male_Female_HandInHand_1/1 -> Actuator/1

== system radar_final_cs_old/Audi_A3_2/SELF_Demux ==
  SELF : Inport  OutDataTypeStr=Bus: PRESCAN_SELFSENSORDATA
  Bus Selector : BusSelector  OutputSignals=PositionX,PositionY,PositionZ,OrientationRoll,OrientationPitch,OrientationYaw,Velocity,Yaw_rate,Lat,Long,Alt,TimeStamp
  Demux2 : Demux  Outputs=3
  Gain : Gain  Gain=180/pi
  Gain1 : Gain  Gain=180/pi
  Vector Concatenate1 : Concatenate  NumInputs=3
  compas converter : Subsystem
  x [m] : Outport
  y [m] : Outport  Port=2
  z [m] : Outport  Port=3
  rotx [deg] : Outport  Port=4
  roty [deg] : Outport  Port=5
  rotz [deg] : Outport  Port=6
  GPS lat [deg] : Outport  Port=7
  GPS long [deg] : Outport  Port=8
  GPS alt [m] : Outport  Port=9
  velocity [m/s] : Outport  Port=10
  heading [deg] : Outport  Port=11
  yaw rate [deg/s] : Outport  Port=12
  TimeStamp [s] : Outport  Port=13
  wires:
  Bus Selector/12 -> TimeStamp [s]/1  "<TimeStamp>"
  Bus Selector/11 -> GPS alt [m]/1  "<Alt>"
  Bus Selector/10 -> GPS long [deg]/1  "<Long>"
  Bus Selector/9 -> GPS lat [deg]/1  "<Lat>"
  Bus Selector/8 -> Gain1/1  "<Yaw_rate>"
  Bus Selector/7 -> velocity [m/s]/1  "<Velocity>"
  Bus Selector/6 -> compas converter/1(rotz [rad]), Vector Concatenate1/3  "<OrientationYaw>"
  Bus Selector/5 -> Vector Concatenate1/2  "<OrientationPitch>"
  Bus Selector/4 -> Vector Concatenate1/1  "<OrientationRoll>"
  Vector Concatenate1/1 -> Gain/1
  Bus Selector/3 -> z [m]/1  "<PositionZ>"
  Bus Selector/2 -> y [m]/1  "<PositionY>"
  Bus Selector/1 -> x [m]/1  "<PositionX>"
  SELF/1 -> Bus Selector/1
  Gain/1 -> Demux2/1
  Demux2/1 -> rotx [deg]/1
  Demux2/2 -> roty [deg]/1
  Demux2/3 -> rotz [deg]/1
  compas converter/1(heading [deg]) -> heading [deg]/1
  Gain1/1 -> yaw rate [deg/s]/1

== system radar_final_cs_old/Boy_150_1/Animation ==
  In1 : Inport
  Bus Creator : BusCreator  Inputs=2  OutDataTypeStr=Bus: PRESCAN_ANIMACTUATORDATA  NonVirtualBus=on
  Bus Selector : BusSelector  OutputSignals=VelocityX,VelocityY,VelocityZ
  Mux : Mux  Inputs=3
  animation mode : Subsystem
  elapsed track : Subsystem
  Out1 : Outport
  wires:
  animation mode/1(mode) -> Bus Creator/1  "Index"
  Bus Creator/1 -> Out1/1
  In1/1 -> Bus Selector/1
  elapsed track/1(s) -> Bus Creator/2  "Time"
  Bus Selector/3 -> Mux/3  "<VelocityZ>"
  Bus Selector/2 -> Mux/2  "<VelocityY>"
  Bus Selector/1 -> Mux/1  "<VelocityX>"
  Mux/1 -> animation mode/1(vel), elapsed track/1(vel)

== system radar_final_cs_old/Boy_150_1/Dynamics_Empty ==
  note: For state mode 'Dynamic' positions
      | are not taken into account, as they
      | are computed by integrating velocity.
      | Click annotation for Help.
  Ground_{1..9} (9 alike) : Ground
  MuxState : Subsystem  Tag=mux/State  mask(Empty Dynamics State Block){positioningmode=on, TimeStep=1/20}
      mask prompts: positioningmode "Positioning Mode"; TimeStep "Auto Assigned: Time Step [s]"
      mask help:
      | Build the state of an actor based on user input.
      | The user can either use positioning mode or dynamics mode.
      | - When using positioning mode the position and orientation of the actor are set directly based on the input. Expected input is relative to the initial position and orientation of the actor. It's also possible to specify the velocity of the actor, though this input isn't used, only passed on.
      | - When using dynamics mode the position input is ignored. Expected input is velocity and orientation. The velocity is relative the current orientation of the actor, while orientation is relative to its initial orientation. The position of the actor is calculated based on the velocity and orientation given.
      settings: DeleteFcn=PreScanBlockDeleteFcn;
  STATE_Boy_150_1 : Subsystem  Tag=mux/StatePort  Priority=0  LoadFcn=load PrescanStateActuatorData  mask(PreScan Sink Block: State){x0=radar_final_cs_Boy_150_1_Dynamics_Empty_STATE_Boy_150_1_x0, y0=radar_final_cs_Boy_150_1_Dynamics_Empty_STATE_Boy_150_1_y0, z0=radar_final_cs_Boy_150_1_Dynamics_Empty_STATE_Boy_150_1_z0, Roll0=radar_final_cs_Boy_150_1_Dynamics_Empty_STATE_Boy_150_1_Roll0, Pitch0=radar_final_cs_Boy_150_1_Dynamics_Empty_STATE_Boy_150_1_Pitch0, Yaw0=radar_final_cs_Boy_150_1_Dynamics_Empty_STATE_Boy_150_1_Yaw0, TimeStep=1/20}
      mask prompts: x0 "Ini x-position VEHICLE wrt GLOBAL axis system [m]"; y0 "Ini y-position VEHICLE wrt GLOBAL axis system [m]"; z0 "Ini z-position VEHICLE wrt GLOBAL axis system [m]"; Roll0 "Ini roll-angle BODY wrt VEHICLE axis system [deg]"; Pitch0 "Ini pitch-angle BODY wrt VEHICLE axis system [deg]"; Yaw0 "Ini yaw-angle VEHICLE wrt GLOBAL axis system [deg]"; TimeStep "Auto-Assigned: Upload Period [s]"
      mask help:
      | The Actor State contains a vector signal of size (9x1), containing the following signals:
      |
      | -  Position                  (x,y,z)                                     [m]
      | -  Velocity                  (vx,vy,vz)                               [m/s]
      | -  Angles                    (Roll, Pitch, Yaw)                   [rad]
      |
      | The Actor state is defined in the global axis system.
      | The state is superponed on the Initial position defined in the GUI.
      |
      | For more information, please click Help.
      settings: DeleteFcn=PreScanBlockDeleteFcn;
      mask Help: eval('openHelp(222)')
      mask Display: image(imread('State.png'))
  State : Outport  Tag=outport/StateOutport  SampleTime=1/20
  wires:
  MuxState/1(state) -> STATE_Boy_150_1/1(State)
  STATE_Boy_150_1/1(StateBus) -> State/1
  Ground_1/1 -> MuxState/1(x [m])
  Ground_2/1 -> MuxState/2(y [m])
  Ground_3/1 -> MuxState/3(z [m])
  Ground_4/1 -> MuxState/4(dx [m/s])
  Ground_5/1 -> MuxState/5(dy [m/s])
  Ground_6/1 -> MuxState/6(dz [m/s])
  Ground_7/1 -> MuxState/7(R [rad])
  Ground_8/1 -> MuxState/8(P [rad])
  Ground_9/1 -> MuxState/9(Y [rad])

== system radar_final_cs_old/Boy_150_1/SELF_Demux ==
  SELF : Inport  OutDataTypeStr=Bus: PRESCAN_SELFSENSORDATA
  Bus Selector : BusSelector  OutputSignals=PositionX,PositionY,PositionZ,OrientationRoll,OrientationPitch,OrientationYaw,Velocity,Yaw_rate,Lat,Long,Alt,TimeStamp
  Demux2 : Demux  Outputs=3
  Gain : Gain  Gain=180/pi
  Gain1 : Gain  Gain=180/pi
  Vector Concatenate1 : Concatenate  NumInputs=3
  compas converter : Subsystem
  x [m] : Outport
  y [m] : Outport  Port=2
  z [m] : Outport  Port=3
  rotx [deg] : Outport  Port=4
  roty [deg] : Outport  Port=5
  rotz [deg] : Outport  Port=6
  GPS lat [deg] : Outport  Port=7
  GPS long [deg] : Outport  Port=8
  GPS alt [m] : Outport  Port=9
  velocity [m/s] : Outport  Port=10
  heading [deg] : Outport  Port=11
  yaw rate [deg/s] : Outport  Port=12
  TimeStamp [s] : Outport  Port=13
  wires:
  Bus Selector/12 -> TimeStamp [s]/1  "<TimeStamp>"
  Bus Selector/11 -> GPS alt [m]/1  "<Alt>"
  Bus Selector/10 -> GPS long [deg]/1  "<Long>"
  Bus Selector/9 -> GPS lat [deg]/1  "<Lat>"
  Bus Selector/8 -> Gain1/1  "<Yaw_rate>"
  Bus Selector/7 -> velocity [m/s]/1  "<Velocity>"
  Bus Selector/6 -> compas converter/1(rotz [rad]), Vector Concatenate1/3  "<OrientationYaw>"
  Bus Selector/5 -> Vector Concatenate1/2  "<OrientationPitch>"
  Bus Selector/4 -> Vector Concatenate1/1  "<OrientationRoll>"
  Vector Concatenate1/1 -> Gain/1
  Bus Selector/3 -> z [m]/1  "<PositionZ>"
  Bus Selector/2 -> y [m]/1  "<PositionY>"
  Bus Selector/1 -> x [m]/1  "<PositionX>"
  SELF/1 -> Bus Selector/1
  Gain/1 -> Demux2/1
  Demux2/1 -> rotx [deg]/1
  Demux2/2 -> roty [deg]/1
  Demux2/3 -> rotz [deg]/1
  compas converter/1(heading [deg]) -> heading [deg]/1
  Gain1/1 -> yaw rate [deg/s]/1

== system radar_final_cs_old/Boy_150_1/VISUColorRegion_Lower_Body_Mux ==
  RGB [-,-,-] : Inport
  Bus Creator : BusCreator  Inputs=4  OutDataTypeStr=Bus: PRESCAN_COLOR_DATA  NonVirtualBus=on
  Constant : Constant  Value=255  OutDataTypeStr=uint8
  Data Type Conversion : DataTypeConversion  OutDataTypeStr=uint8
  Data Type Conversion1 : DataTypeConversion  OutDataTypeStr=uint8
  Data Type Conversion2 : DataTypeConversion  OutDataTypeStr=uint8
  Demux : Demux  Outputs=3
  ColorRegion : Outport  OutDataTypeStr=Bus: PRESCAN_COLOR_DATA  PortDimensions=1
  wires:
  Constant/1 -> Bus Creator/4  "A"
  Data Type Conversion2/1 -> Bus Creator/3  "B"
  Data Type Conversion1/1 -> Bus Creator/2  "G"
  Data Type Conversion/1 -> Bus Creator/1  "R"
  Demux/3 -> Data Type Conversion2/1  "B"
  Demux/2 -> Data Type Conversion1/1  "G"
  Demux/1 -> Data Type Conversion/1  "R"
  RGB [-,-,-]/1 -> Demux/1
  Bus Creator/1 -> ColorRegion/1

== system radar_final_cs_old/Boy_150_1/VISUColorRegion_Shoes_Mux ==
  RGB [-,-,-] : Inport
  Bus Creator : BusCreator  Inputs=4  OutDataTypeStr=Bus: PRESCAN_COLOR_DATA  NonVirtualBus=on
  Constant : Constant  Value=255  OutDataTypeStr=uint8
  Data Type Conversion : DataTypeConversion  OutDataTypeStr=uint8
  Data Type Conversion1 : DataTypeConversion  OutDataTypeStr=uint8
  Data Type Conversion2 : DataTypeConversion  OutDataTypeStr=uint8
  Demux : Demux  Outputs=3
  ColorRegion : Outport  OutDataTypeStr=Bus: PRESCAN_COLOR_DATA  PortDimensions=1
  wires:
  Constant/1 -> Bus Creator/4  "A"
  Data Type Conversion2/1 -> Bus Creator/3  "B"
  Data Type Conversion1/1 -> Bus Creator/2  "G"
  Data Type Conversion/1 -> Bus Creator/1  "R"
  Demux/3 -> Data Type Conversion2/1  "B"
  Demux/2 -> Data Type Conversion1/1  "G"
  Demux/1 -> Data Type Conversion/1  "R"
  RGB [-,-,-]/1 -> Demux/1
  Bus Creator/1 -> ColorRegion/1

== system radar_final_cs_old/Boy_150_1/VISUColorRegion_Upper_Body_Mux ==
  RGB [-,-,-] : Inport
  Bus Creator : BusCreator  Inputs=4  OutDataTypeStr=Bus: PRESCAN_COLOR_DATA  NonVirtualBus=on
  Constant : Constant  Value=255  OutDataTypeStr=uint8
  Data Type Conversion : DataTypeConversion  OutDataTypeStr=uint8
  Data Type Conversion1 : DataTypeConversion  OutDataTypeStr=uint8
  Data Type Conversion2 : DataTypeConversion  OutDataTypeStr=uint8
  Demux : Demux  Outputs=3
  ColorRegion : Outport  OutDataTypeStr=Bus: PRESCAN_COLOR_DATA  PortDimensions=1
  wires:
  Constant/1 -> Bus Creator/4  "A"
  Data Type Conversion2/1 -> Bus Creator/3  "B"
  Data Type Conversion1/1 -> Bus Creator/2  "G"
  Data Type Conversion/1 -> Bus Creator/1  "R"
  Demux/3 -> Data Type Conversion2/1  "B"
  Demux/2 -> Data Type Conversion1/1  "G"
  Demux/1 -> Data Type Conversion/1  "R"
  RGB [-,-,-]/1 -> Demux/1
  Bus Creator/1 -> ColorRegion/1

== system radar_final_cs_old/Child_Leaning_1/Dynamics_Empty ==
  note: For state mode 'Dynamic' positions
      | are not taken into account, as they
      | are computed by integrating velocity.
      | Click annotation for Help.
  Ground_{1..9} (9 alike) : Ground
  MuxState : Subsystem  Tag=mux/State  mask(Empty Dynamics State Block){positioningmode=on, TimeStep=1/20}
      mask prompts: positioningmode "Positioning Mode"; TimeStep "Auto Assigned: Time Step [s]"
      mask help:
      | Build the state of an actor based on user input.
      | The user can either use positioning mode or dynamics mode.
      | - When using positioning mode the position and orientation of the actor are set directly based on the input. Expected input is relative to the initial position and orientation of the actor. It's also possible to specify the velocity of the actor, though this input isn't used, only passed on.
      | - When using dynamics mode the position input is ignored. Expected input is velocity and orientation. The velocity is relative the current orientation of the actor, while orientation is relative to its initial orientation. The position of the actor is calculated based on the velocity and orientation given.
      settings: DeleteFcn=PreScanBlockDeleteFcn;
  STATE_Child_Leaning_1 : Subsystem  Tag=mux/StatePort  Priority=0  LoadFcn=load PrescanStateActuatorData  mask(PreScan Sink Block: State){x0=radar_final_cs_bd2c14ed7a8a21e4, y0=radar_final_cs_2a9ff95eb5b29c63, z0=radar_final_cs_25fb437f13dc4ac4, Roll0=radar_final_cs_647e288b34857263, Pitch0=radar_final_cs_57cb0909d4e1963a, Yaw0=radar_final_cs_bdb595cdc91a90da, TimeStep=1/20}
      mask prompts: x0 "Ini x-position VEHICLE wrt GLOBAL axis system [m]"; y0 "Ini y-position VEHICLE wrt GLOBAL axis system [m]"; z0 "Ini z-position VEHICLE wrt GLOBAL axis system [m]"; Roll0 "Ini roll-angle BODY wrt VEHICLE axis system [deg]"; Pitch0 "Ini pitch-angle BODY wrt VEHICLE axis system [deg]"; Yaw0 "Ini yaw-angle VEHICLE wrt GLOBAL axis system [deg]"; TimeStep "Auto-Assigned: Upload Period [s]"
      mask help:
      | The Actor State contains a vector signal of size (9x1), containing the following signals:
      |
      | -  Position                  (x,y,z)                                     [m]
      | -  Velocity                  (vx,vy,vz)                               [m/s]
      | -  Angles                    (Roll, Pitch, Yaw)                   [rad]
      |
      | The Actor state is defined in the global axis system.
      | The state is superponed on the Initial position defined in the GUI.
      |
      | For more information, please click Help.
      settings: DeleteFcn=PreScanBlockDeleteFcn;
      mask Help: eval('openHelp(222)')
      mask Display: image(imread('State.png'))
  State : Outport  Tag=outport/StateOutport  SampleTime=1/20
  wires:
  MuxState/1(state) -> STATE_Child_Leaning_1/1(State)
  STATE_Child_Leaning_1/1(StateBus) -> State/1
  Ground_1/1 -> MuxState/1(x [m])
  Ground_2/1 -> MuxState/2(y [m])
  Ground_3/1 -> MuxState/3(z [m])
  Ground_4/1 -> MuxState/4(dx [m/s])
  Ground_5/1 -> MuxState/5(dy [m/s])
  Ground_6/1 -> MuxState/6(dz [m/s])
  Ground_7/1 -> MuxState/7(R [rad])
  Ground_8/1 -> MuxState/8(P [rad])
  Ground_9/1 -> MuxState/9(Y [rad])

== system radar_final_cs_old/Child_Leaning_1/SELF_Demux ==
  SELF : Inport  OutDataTypeStr=Bus: PRESCAN_SELFSENSORDATA
  Bus Selector : BusSelector  OutputSignals=PositionX,PositionY,PositionZ,OrientationRoll,OrientationPitch,OrientationYaw,Velocity,Yaw_rate,Lat,Long,Alt,TimeStamp
  Demux2 : Demux  Outputs=3
  Gain : Gain  Gain=180/pi
  Gain1 : Gain  Gain=180/pi
  Vector Concatenate1 : Concatenate  NumInputs=3
  compas converter : Subsystem
  x [m] : Outport
  y [m] : Outport  Port=2
  z [m] : Outport  Port=3
  rotx [deg] : Outport  Port=4
  roty [deg] : Outport  Port=5
  rotz [deg] : Outport  Port=6
  GPS lat [deg] : Outport  Port=7
  GPS long [deg] : Outport  Port=8
  GPS alt [m] : Outport  Port=9
  velocity [m/s] : Outport  Port=10
  heading [deg] : Outport  Port=11
  yaw rate [deg/s] : Outport  Port=12
  TimeStamp [s] : Outport  Port=13
  wires:
  Bus Selector/12 -> TimeStamp [s]/1  "<TimeStamp>"
  Bus Selector/11 -> GPS alt [m]/1  "<Alt>"
  Bus Selector/10 -> GPS long [deg]/1  "<Long>"
  Bus Selector/9 -> GPS lat [deg]/1  "<Lat>"
  Bus Selector/8 -> Gain1/1  "<Yaw_rate>"
  Bus Selector/7 -> velocity [m/s]/1  "<Velocity>"
  Bus Selector/6 -> compas converter/1(rotz [rad]), Vector Concatenate1/3  "<OrientationYaw>"
  Bus Selector/5 -> Vector Concatenate1/2  "<OrientationPitch>"
  Bus Selector/4 -> Vector Concatenate1/1  "<OrientationRoll>"
  Vector Concatenate1/1 -> Gain/1
  Bus Selector/3 -> z [m]/1  "<PositionZ>"
  Bus Selector/2 -> y [m]/1  "<PositionY>"
  Bus Selector/1 -> x [m]/1  "<PositionX>"
  SELF/1 -> Bus Selector/1
  Gain/1 -> Demux2/1
  Demux2/1 -> rotx [deg]/1
  Demux2/2 -> roty [deg]/1
  Demux2/3 -> rotz [deg]/1
  compas converter/1(heading [deg]) -> heading [deg]/1
  Gain1/1 -> yaw rate [deg/s]/1

== system radar_final_cs_old/Child_Leaning_1/VISUColorRegion_Lower_Body_Mux ==
  RGB [-,-,-] : Inport
  Bus Creator : BusCreator  Inputs=4  OutDataTypeStr=Bus: PRESCAN_COLOR_DATA  NonVirtualBus=on
  Constant : Constant  Value=255  OutDataTypeStr=uint8
  Data Type Conversion : DataTypeConversion  OutDataTypeStr=uint8
  Data Type Conversion1 : DataTypeConversion  OutDataTypeStr=uint8
  Data Type Conversion2 : DataTypeConversion  OutDataTypeStr=uint8
  Demux : Demux  Outputs=3
  ColorRegion : Outport  OutDataTypeStr=Bus: PRESCAN_COLOR_DATA  PortDimensions=1
  wires:
  Constant/1 -> Bus Creator/4  "A"
  Data Type Conversion2/1 -> Bus Creator/3  "B"
  Data Type Conversion1/1 -> Bus Creator/2  "G"
  Data Type Conversion/1 -> Bus Creator/1  "R"
  Demux/3 -> Data Type Conversion2/1  "B"
  Demux/2 -> Data Type Conversion1/1  "G"
  Demux/1 -> Data Type Conversion/1  "R"
  RGB [-,-,-]/1 -> Demux/1
  Bus Creator/1 -> ColorRegion/1
